simulink model "lab1"  (R2020b)
settings: Solver=VariableStepAuto  StartTime=0.0  StopTime=10.0  RelTol=1e-3
settings Model: Creator=FORVARD  LastModifiedBy=FORVARD

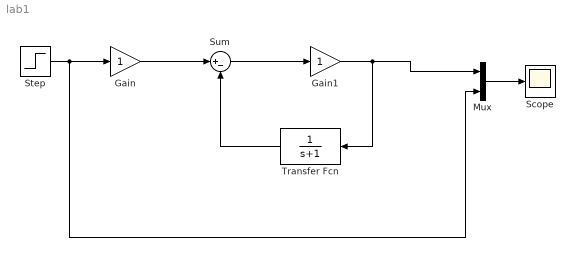
== system lab1 ==
  Gain : Gain
  Gain1 : Gain
  Mux : Mux  Inputs=2
  Scope : Scope
  Step : Step  Time=0  SampleTime=0
  Sum : Sum  Inputs=|+-
  Transfer Fcn : TransferFcn  Denominator=[1 1]
  wires:
  Step/1 -> Gain/1, Mux/2
  Mux/1 -> Scope/1
  Gain/1 -> Sum/1
  Sum/1 -> Gain1/1
  Gain1/1 -> Transfer Fcn/1, Mux/1
  Transfer Fcn/1 -> Sum/2
